simulink model "vrmorph"  (Simulink 7.5)
settings: Solver=VariableStepDiscrete  StartTime=0.0  StopTime=Inf  RelTol=1e-3
libraries: simulink x1, vrlib x1
Description:
  | Geometry Morphing
  | 
  | This example shows how the VR Sink block
  | accepts matrix signals and variable-size signals.
  | We modify the vertex coordinates of a block
  | resulting in the change of the object's shape.
  | 
  | The manual switch allows to switch between
  | rendering the whole object and its upper half,
  | showing how input signal dimensions can
  | change while the simulation runs.
settings Model: Creator=Stepanek  LastModifiedBy=Houska
settings SolverCC: InsertRTBMode=Auto
settings OptimizationCC: InitFltsAndDblsToZero=on
settings DebuggingCC: SolverPrmCheckMsg=none  StrictBusMsg=Warning

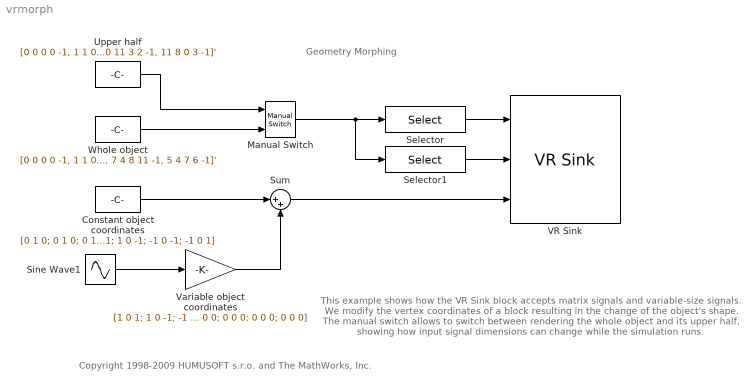
== system vrmorph ==
  note: Copyright 1998-2009 HUMUSOFT s.r.o. and The MathWorks, Inc.
  note: This example shows how the VR Sink block
      | accepts matrix signals and variable-size signals.
      | We modify the vertex coordinates of a block
      | resulting in the change of the object's shape.
      |
      | The manual switch allows to switch between
      | rendering the whole object and its upper half,
      | showing how input signal dimensions can
      | change while the simulation runs.
  note: Geometry Morphing
  Constant object coordinates : Constant  Value=[0 1 0; 0 1 0; 0 1 0; 0 1 0; 0 -1 0; 0 -1 0; 0 -1 0; 0 -1 0; 1 0 1; 1 0 -1; -1 0 -1; -1 0 1]  OutDataType=sfix(16)  OutScaling=2^0
  Manual Switch : simulink/Signal Routing/Manual Switch  SystemSampleTime=-1  sw=0  action=0  varsize=on
  Selector : Selector  NumberOfDimensions=2  InputPortWidth=3  IndexOptions=Select all,Index vector (dialog)  Indices=[1 3],1  OutputSizes=1,1
  Selector1 : Selector  NumberOfDimensions=2  InputPortWidth=3  IndexOptions=Select all,Index vector (dialog)  Indices=[1 3],2  OutputSizes=1,1
  Sine Wave1 : Sin  Amplitude=0.5  Bias=0.5  Frequency=0.2  Phase=pi/2  Samples=10  SampleTime=0  Offset=0
  Sum : Sum  Inputs=|++  OutDataType=sfix(16)  OutScaling=2^0
  Upper half : Constant  Value=[0 0 0 0 -1, 1 1 0 0 -1, 1 2 0 0 -1, 2 3 0 0 -1, 3 1 0 0 -1; 0 1 2 3 -1, 8 9 1 0 -1, 9 10 2 1 -1, 10 11 3 2 -1, 11 8 0 3 -1]'  VectorParams1D=off  OutDataType=sfix(16)  OutScaling=2^0
  VR Sink : vrlib/VR Sink  InstantiateOnLoad=on  SampleTime=0.1  ViewEnable=on  RemoteChange=off  RemoteView=on  FieldsWritten=IFS.colorIndex.1.-1.1.double#IFS.coordIndex.1.-1.1.double#IFS_Coords.point.3.-1.1.double  WorldFileName=vrmorph.wrl  WorldDescription=VR Geometry Morphing  AutoView=on  VideoDimensions=[]  FigureProperties="{'Position', 'Name', 'Viewpoint', 'CameraBound', 'CameraDirection', 'CameraPosition', 'CameraUpVector', 'ZoomFactor', 'Antialiasing', 'Headlight', 'Lighting', 'NavPanel', 'StatusBar', 'ToolBar', 'Textures', 'Transparency', 'Wireframe', 'NavZones', 'NavMode', 'NavSpeed', 'Record2DCompressMethod', 'Record2DCompressQuality', 'Record2D', 'Record2DFileName', 'Record2DFPS'; [1.1000000000000000e+001  7.8000000000000000e+001  4.9300000000000000e+002  3.6800000000000000e+002], 'VR Geometry Morphing', 'View 1', 'on', [0.0000000000000000e+000  0.0000000000000000e+000 -1.0000000000000000e+000], [0.0000000000000000e+000  0.0000000000000000e+000  0.0000000000000000e+000], [0.0000000000000000e+000  1.0000000000000000e+000  0.0000000000000000e+000], [1.0000000000000000e+000], 'off', 'on', 'on', 'halfbar', 'on', 'on', 'on', 'on', 'off', 'off', 'examine', 'normal', 'auto', [7.5000000000000000e+001], 'off', '%f_anim_%n.avi', [1.5000000000000000e+001]}"
  Variable object coordinates : Gain  Gain=[1 0 1; 1 0 -1; -1 0 -1; -1 0 1; 1 0 1; 1 0 -1; -1 0 -1; -1 0 1; 0 0 0; 0 0 0; 0 0 0; 0 0 0]  ParameterDataType=sfix(16)  ParameterScaling=2^0  OutDataType=sfix(16)  OutScaling=2^0
  Whole object : Constant  Value=[0 0 0 0 -1, 1 1 0 0 -1, 1 2 0 0 -1, 2 3 0 0 -1, 3 1 0 0 -1, 4 4 1 1 -1, 4 4 2 1 -1, 4 4 3 2 -1, 4 4 1 3 -1, 4 4 4 4 -1; 0 1 2 3 -1, 8 9 1 0 -1, 9 10 2 1 -1, 10 11 3 2 -1, 11 8 0 3 -1, 4 5 9 8 -1, 5 6 10 9 -1, 6 7 11 10 -1, 7 4 8 11 -1, 5 4 7 6 -1]'  VectorParams1D=off  OutDataType=sfix(16)  OutScaling=2^0
  wires:
  Upper half/1 -> Manual Switch/1
  Whole object/1 -> Manual Switch/2
  Selector/1 -> VR Sink/1
  Selector1/1 -> VR Sink/2
  Variable object coordinates/1 -> Sum/2
  Constant object coordinates/1 -> Sum/1
  Sine Wave1/1 -> Variable object coordinates/1
  Sum/1 -> VR Sink/3
  Manual Switch/1 -> Selector/1, Selector1/1
